simulink model "Sim_PID_01"  (R2020b)
settings: Solver=FixedStepAuto  StartTime=0.0  StopTime=simtime  FixedStep=1/CF  RelTol=1e-3
InitFcn:
  | PID_startup
values from neighbouring files (symbols this model uses):
  BLS = a^2*(Bm + Bt) + Bg    (= 0.00020001)    [PID_startup.m]
  CF = 500    [PID_startup.m]
  JLS = a^2*(Jm+Jp) + Jg + Jl    (= 0.00110051)    [PID_startup.m]
  K = 1    [PID_startup.m]
  Kd = 5    [PID_startup.m]
  Ki = 2    [PID_startup.m]
  Km = 6.95e-3    (= 0.00695)    [PID_startup.m]
  Kp = 2    [PID_startup.m]
  L = 1.8e-3    (= 0.0018)    [PID_startup.m]
  R = 2    [PID_startup.m]
  Sg = 1    [PID_startup.m]
settings Model: Creator=miyaz  LastModifiedBy=miyaz

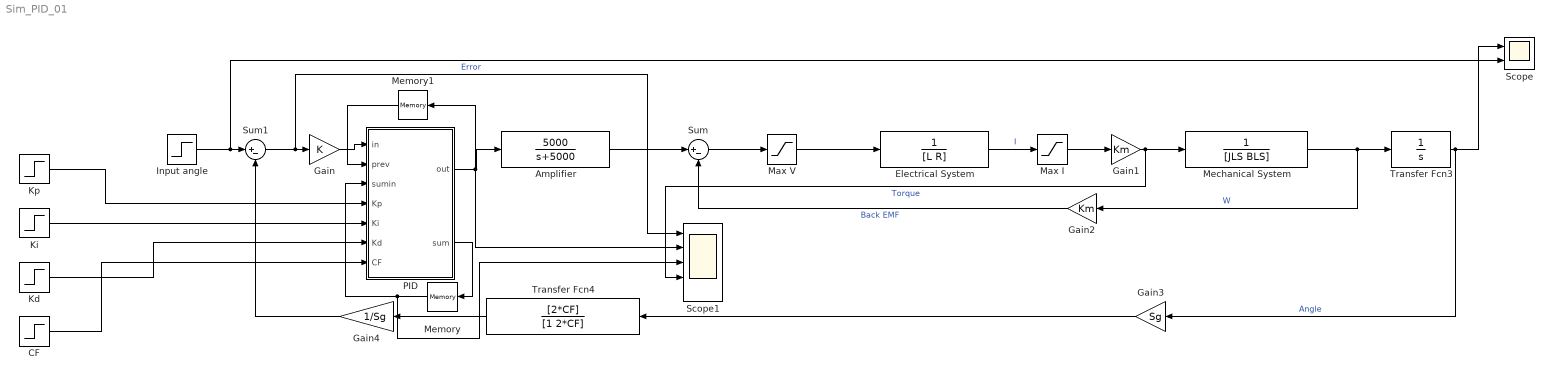
== system Sim_PID_01 ==
  Amplifier : TransferFcn  Numerator=[5000]  Denominator=[1 5000]
  CF : Step  Time=0  After=CF  SampleTime=0
  Electrical System : TransferFcn  Denominator=[L R]
  Gain : Gain  Gain=K
  Gain1 : Gain  Gain=Km
  Gain2 : Gain  Gain=Km
  Gain3 : Gain  Gain=Sg
  Gain4 : Gain  Gain=1/Sg
  Input angle : Step  After=pi/2  SampleTime=0
  Kd : Step  Time=0  After=Kd  SampleTime=0
  Ki : Step  Time=0  After=Ki  SampleTime=0
  Kp : Step  Time=0  After=Kp  SampleTime=0
  Max I : Saturate  UpperLimit=5  LowerLimit=-5
  Max V : Saturate  UpperLimit=50  LowerLimit=-50
  Mechanical System : TransferFcn  Denominator=[JLS BLS]
  Memory : Memory  InheritSampleTime=on
  Memory1 : Memory  InheritSampleTime=on
  PID : MATLAB Function  TreatAsAtomicUnit=on
  Scope : Scope  NumInputPorts=2
  Scope1 : Scope  NumInputPorts=5
  Sum : Sum  Inputs=|+-
  Sum1 : Sum  Inputs=|+-
  Transfer Fcn3 : TransferFcn  Denominator=[1 0]
  Transfer Fcn4 : TransferFcn  Numerator=[2*CF]  Denominator=[1 2*CF]
  wires:
  Input angle/1 -> Sum1/1, Scope/2
  Sum1/1 -> Scope1/1, Gain/1  "Error"
  Transfer Fcn3/1 -> Gain3/1, Scope/1  "Angle"
  Mechanical System/1 -> Gain2/1, Transfer Fcn3/1  "W"
  Gain1/1 -> Scope1/4, Mechanical System/1  "Torque"
  Gain2/1 -> Sum/2  "Back EMF"
  Gain3/1 -> Transfer Fcn4/1
  Gain/1 -> PID/1(in)
  PID/1(out) -> Memory1/1, Amplifier/1, Scope1/2
  Gain4/1 -> Sum1/2
  Transfer Fcn4/1 -> Gain4/1
  PID/2(sum) -> Memory/1
  Kp/1 -> PID/4(Kp)
  Ki/1 -> PID/5(Ki)
  Kd/1 -> PID/6(Kd)
  CF/1 -> PID/7(CF)
  Memory/1 -> Scope1/3, PID/3(sumin)
  Memory1/1 -> PID/2(prev)
  Max I/1 -> Gain1/1
  Electrical System/1 -> Max I/1  "I"
  Amplifier/1 -> Sum/1
  Sum/1 -> Max V/1
  Max V/1 -> Electrical System/1

== matlab function Sim_PID_01/PID ==
  data: in input; out output; prev input; sum output; sumin input; Kp input; Ki input; Kd input; CF input
function [out, sum] = fcn(in, prev, sumin, Kp ,Ki ,Kd ,CF)
out = Kp*in + Ki*(in + sumin)+Kd*(in-prev)/(1/CF);
sum = in+sumin;
